simulink model "exemplo1sim"  (R2024a)
settings: Solver=ode4  StartTime=0.0  StopTime=10.0  RelTol=1e-3
values from neighbouring files (symbols this model uses):
  e0 = [1; 0; 0]    [exemplo1.m]
  K = acker(A, B, mus)    [exemplo1.m]
  Ke = acker(sys_dual.A, sys_dual.B, po)'    [exemplo1.m]
undefined symbols (not defined in the file or in its folder): A, B, C
settings Model: Creator=caugu  LastModifiedBy=caugu

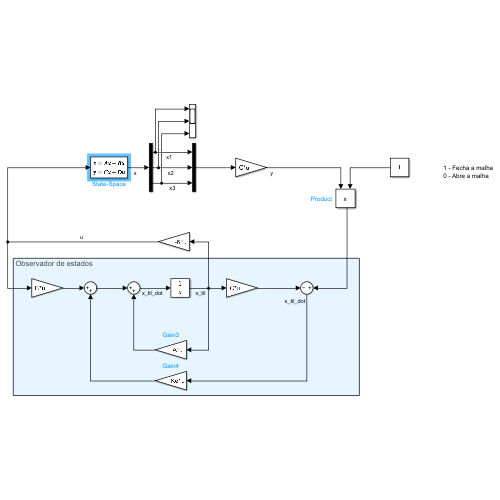
[thumbnail: Simulink's stored preview of the top-level diagram]
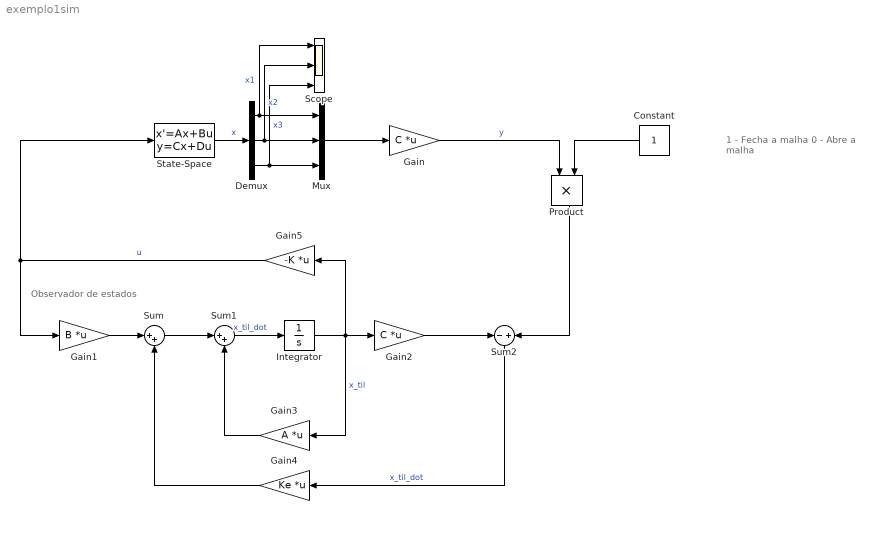
== system exemplo1sim ==
  note: Observador de estados
  note: 1 - Fecha a malha
      | 0 - Abre a malha
  Constant : Constant
  Demux : Demux  Outputs=3
  Gain : Gain  Gain=C  Multiplication=Matrix(K*u)
  Gain1 : Gain  Gain=B  Multiplication=Matrix(K*u)
  Gain2 : Gain  Gain=C  Multiplication=Matrix(K*u)
  Gain3 : Gain  Gain=A  Multiplication=Matrix(K*u)
  Gain4 : Gain  Gain=Ke  Multiplication=Matrix(K*u)
  Gain5 : Gain  Gain=-K  Multiplication=Matrix(K*u)
  Integrator : Integrator  InitialCondition=e0
  Mux : Mux  Inputs=3
  Product : Product
  Scope : Scope  NumInputPorts=3
  State-Space : StateSpace  InitialCondition=0
  Sum : Sum  Inputs=|++
  Sum1 : Sum  Inputs=|++
  Sum2 : Sum  Inputs=-+
  wires:
  Demux/1 -> Scope/1, Mux/1  "x1"
  Demux/3 -> Scope/3, Mux/3  "x3"
  Demux/2 -> Scope/2, Mux/2  "x2"
  State-Space/1 -> Demux/1  "x"
  Mux/1 -> Gain/1
  Gain1/1 -> Sum/1
  Sum/1 -> Sum1/1
  Sum1/1 -> Integrator/1  "x_til_dot"
  Integrator/1 -> Gain5/1, Gain3/1, Gain2/1  "x_til"
  Gain2/1 -> Sum2/1
  Gain3/1 -> Sum1/2
  Gain4/1 -> Sum/2
  Sum2/1 -> Gain4/1  "x_til_dot"
  Gain5/1 -> Gain1/1, State-Space/1  "u"
  Gain/1 -> Product/1  "y"
  Product/1 -> Sum2/2
  Constant/1 -> Product/2
